simulink model "Exp_5_problem_3"  (R2022b)
settings: Solver=VariableStepAuto  StartTime=0.0  StopTime=10.0  RelTol=1e-3
settings Model: Creator=HP  LastModifiedBy=HP

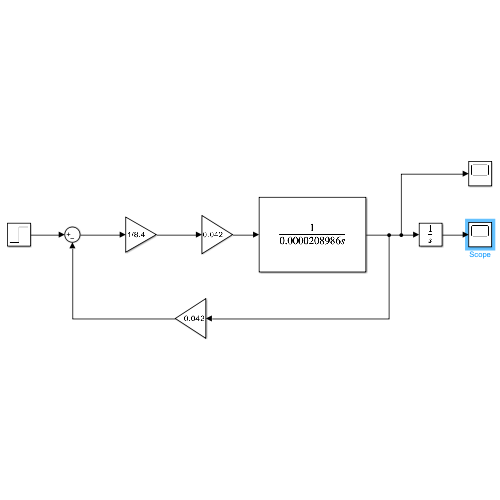
[thumbnail: Simulink's stored preview of the top-level diagram]
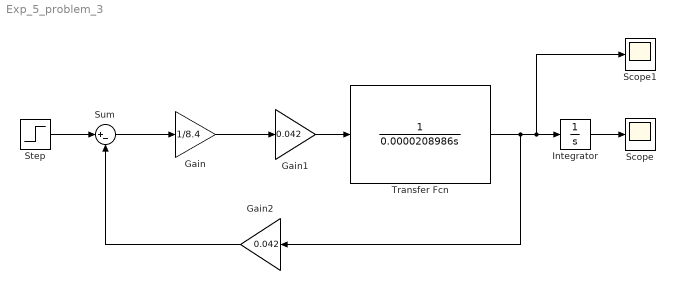
== system Exp_5_problem_3 ==
  Gain : Gain  Gain=1/8.4  RndMeth=Round
  Gain1 : Gain  Gain=0.042
  Gain2 : Gain  Gain=0.042
  Integrator : Integrator
  Scope : Scope
  Scope1 : Scope
  Step : Step  SampleTime=0
  Sum : Sum  Inputs=|+-
  Transfer Fcn : TransferFcn  Denominator=[0.0000208986 0]
  wires:
  Step/1 -> Sum/1
  Sum/1 -> Gain/1
  Gain/1 -> Gain1/1
  Gain1/1 -> Transfer Fcn/1
  Gain2/1 -> Sum/2
  Transfer Fcn/1 -> Scope1/1, Integrator/1, Gain2/1
  Integrator/1 -> Scope/1
